simulink model "outerLoop_voltageControl"  (R2023b)
settings: Solver=ode1  StartTime=0.0  StopTime=Tsim_outLoop  FixedStep=Tstep  RelTol=1e-3
values from neighbouring files (symbols this model uses):
  C = 1000e-6    (= 0.001)    [DCDC_param.m]
  ILmax = 10    [DCDC_param.m]
  ILnom = 5    [DCDC_param.m]
  ResrC = 1.8e-3    (= 0.0018)    [DCDC_param.m]
  Tsw = 1/fsw    (= 0.0001)    [DCDC_param.m]    (also in adcpwm_setup.m)
  VinNom = 30    [DCDC_param.m]
  VoutNom = 50    [DCDC_param.m]
undefined symbols (not defined in the file or in its folder): den_i, kaw_v, ki_v, kp_v, kpf_v, num_i
settings Model: Creator=nicholas  LastModifiedBy=nicholas

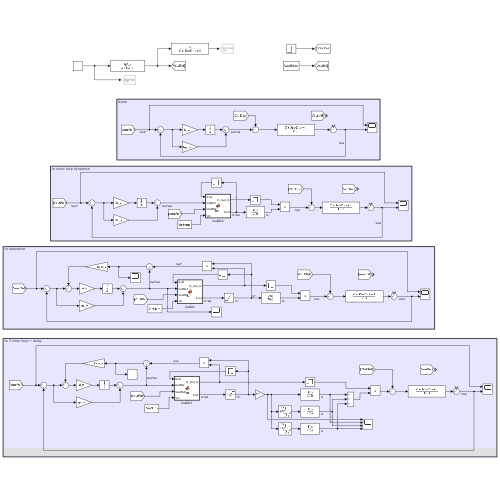
[thumbnail: Simulink's stored preview of the top-level diagram]
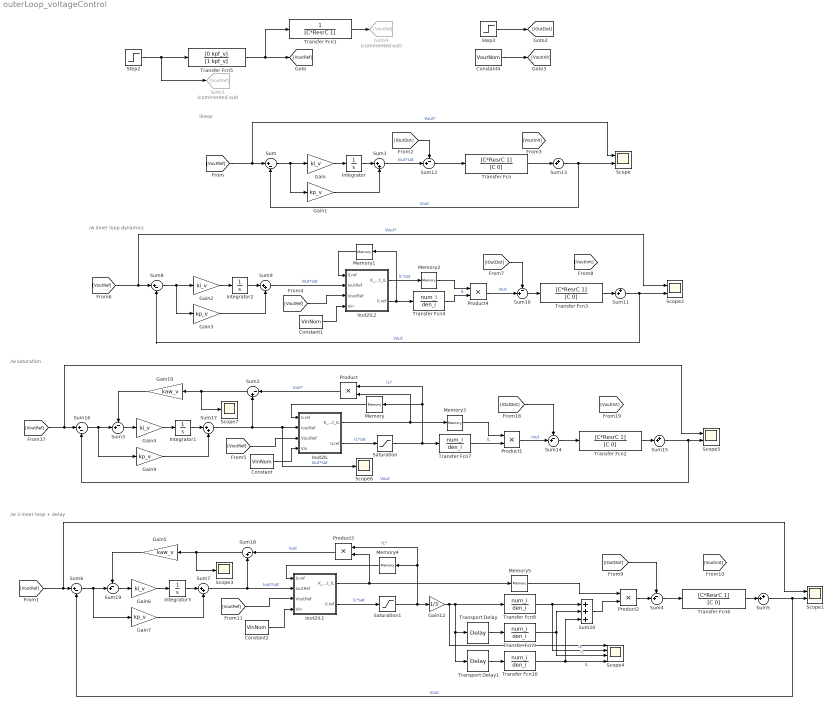
== system outerLoop_voltageControl ==
  note: /w 3 inner loop + delay
  note: /w saturation
  note: /w inner loop dynamics
  note: linear
  Constant : Constant  Value=VinNom
  Constant1 : Constant  Value=VinNom
  Constant2 : Constant  Value=VinNom
  Constant4 : Constant  Value=VoutNom
  Gain{,2,4,6} (4 alike) : Gain  Gain=ki_v
  Gain{1,3,7,9} (4 alike) : Gain  Gain=kp_v
  Gain10 : Gain  Gain=kaw_v
  Gain12 : Gain  Gain=1/3
  Gain5 : Gain  Gain=kaw_v
  Goto1 : Goto  Commented=on  GotoTag=VoutRef
  Goto4 : Goto  Commented=on  GotoTag=VoutRef
  Integrator{,1..3} (4 alike) : Integrator
  Iout2IL : MATLAB Function  TreatAsAtomicUnit=on
  Iout2IL1 : MATLAB Function  TreatAsAtomicUnit=on
  Iout2IL2 : MATLAB Function  TreatAsAtomicUnit=on
  Memory : Memory
  Memory1 : Memory
  Memory2 : Memory  InitialCondition=1
  Memory3 : Memory  InitialCondition=1
  Memory4 : Memory
  Memory5 : Memory  InitialCondition=1
  Product{,1..4} (5 alike) : Product
  Saturation : Saturate  UpperLimit=ILmax  LowerLimit=-ILmax
  Saturation1 : Saturate  UpperLimit=ILmax  LowerLimit=-ILmax
  Scope{,1..2,5} (4 alike) : Scope  NumInputPorts=2
  Scope3 : Scope
  Scope4 : Scope  NumInputPorts=4
  Scope6 : Scope
  Scope7 : Scope
  Step2 : Step  Time=0.1  Before=VinNom  After=VoutNom  SampleTime=0
  Step3 : Step  Time=0.3  After=ILnom/3  SampleTime=0
  Sum{,6,8,16} (4 alike) : Sum  Inputs=|+-
  Sum{1,7,9,17} (4 alike) : Sum  Inputs=|++
  Sum{3..4,10,12,14,19} (6 alike) : Sum  Inputs=-+|
  Sum{5,11,13,15} (4 alike) : Sum  Inputs=++|
  Sum18 : Sum  Inputs=|-+
  Sum2 : Sum  Inputs=|-+
  Sum20 : Sum  Inputs=+++
  Transfer Fcn{,2..3,6} (4 alike) : TransferFcn  Numerator=[C*ResrC 1]  Denominator=[C 0]
  Transfer Fcn1 : TransferFcn  Denominator=[C*ResrC 1]
  Transfer Fcn{4,7..10} (5 alike) : TransferFcn  Numerator=num_i  Denominator=den_i
  Transfer Fcn5 : TransferFcn  Numerator=[0 kpf_v]  Denominator=[1 kpf_v]
  Transport Delay : TransportDelay  DelayTime=Tsw/3
  Transport Delay1 : TransportDelay  DelayTime=2*Tsw/3
  wires:
  [VoutRef] -> Scope/1, Sum/1  "Vout*"
  Gain1/1 -> Sum1/2
  Sum/1 -> Gain/1, Gain1/1
  Gain/1 -> Integrator/1
  Integrator/1 -> Sum1/1
  Sum12/1 -> Transfer Fcn/1
  Step3/1 -> [IOutDist]
  Constant4/1 -> [VoutInit]
  Sum1/1 -> Sum12/2  "Iout*sat"
  Transfer Fcn/1 -> Sum13/2
  Sum13/1 -> Sum/2, Scope/2  "Vout"
  [IOutDist] -> Sum12/1
  Transfer Fcn1/1 -> Goto4/1
  Sum11/1 -> Sum8/2, Scope2/2  "Vout"
  Gain3/1 -> Sum9/2
  Transfer Fcn3/1 -> Sum11/2
  Sum8/1 -> Gain2/1, Gain3/1
  Sum10/1 -> Transfer Fcn3/1
  [VoutRef] -> Scope2/1, Sum8/1  "Vout*"
  Integrator2/1 -> Sum9/1
  [IOutDist] -> Sum10/1
  Gain2/1 -> Integrator2/1
  Product1/1 -> Sum14/2  "Iout"
  Gain9/1 -> Sum17/2
  Sum16/1 -> Sum3/2, Gain9/1
  Sum14/1 -> Transfer Fcn2/1
  Transfer Fcn2/1 -> Sum15/2
  Sum15/1 -> Sum16/2, Scope5/2  "Vout"
  [VoutRef] -> Scope5/1, Sum16/1
  Sum17/1 -> Sum2/2, Scope6/1, Iout2IL/2(IoutRef)  "Iout*sat"
  Integrator1/1 -> Sum17/1
  Sum3/1 -> Gain4/1
  Iout2IL/1(K_Iout_IL) -> Product/2, Memory3/1
  Memory/1 -> Iout2IL/1("ILref ")
  Constant/1 -> Iout2IL/4(Vin)
  Saturation/1 -> Transfer Fcn7/1, Product/1, Memory/1  "IL*"
  Sum9/1 -> Iout2IL2/2(IoutRef)  "Iout*sat"
  Iout2IL2/2(ILref) -> Memory1/1, Transfer Fcn4/1  "IL*sat"
  Memory1/1 -> Iout2IL2/1("ILref ")
  Constant1/1 -> Iout2IL2/4(Vin)
  [VoutRef] -> Iout2IL2/3(VoutRef)
  Product/1 -> Sum2/1  "Iout*"
  Sum2/1 -> Scope7/1, Gain10/1
  Transfer Fcn4/1 -> Product4/2  "IL"
  Product4/1 -> Sum10/2  "Iout"
  Iout2IL2/1(K_Iout_IL) -> Memory2/1
  Memory2/1 -> Product4/1
  Transfer Fcn7/1 -> Product1/2  "IL"
  Memory3/1 -> Product1/1
  Transfer Fcn5/1 -> Transfer Fcn1/1, [VoutRef]
  Step2/1 -> Transfer Fcn5/1, Goto1/1
  Gain4/1 -> Integrator1/1
  Gain10/1 -> Sum3/1
  [VoutRef] -> Iout2IL/3(VoutRef)
  Iout2IL/2(ILref) -> Saturation/1  "IL*sat"
  Integrator3/1 -> Sum7/1
  [VoutRef] -> Iout2IL1/3(VoutRef)
  Saturation1/1 -> Product3/1, Memory4/1, Gain12/1  "IL*"
  Gain6/1 -> Integrator3/1
  Sum7/1 -> Iout2IL1/2(IoutRef), Sum18/2  "Iout*sat"
  [IOutDist] -> Sum4/1
  Gain7/1 -> Sum7/2
  Sum4/1 -> Transfer Fcn6/1
  Iout2IL1/2(ILref) -> Saturation1/1  "IL*sat"
  Product2/1 -> Sum4/2
  Memory5/1 -> Product2/1
  Constant2/1 -> Iout2IL1/4(Vin)
  Sum6/1 -> Sum19/2, Gain7/1
  Iout2IL1/1(K_Iout_IL) -> Product3/2, Memory5/1
  Gain5/1 -> Sum19/1
  Sum5/1 -> Sum6/2, Scope1/2  "Vout"
  Sum19/1 -> Gain6/1
  Sum18/1 -> Scope3/1, Gain5/1
  Memory4/1 -> Iout2IL1/1("ILref ")
  [VoutRef] -> Scope1/1, Sum6/1
  Transfer Fcn6/1 -> Sum5/2
  Product3/1 -> Sum18/1  "Iout"
  Transport Delay/1 -> Transfer Fcn9/1
  Transport Delay1/1 -> Transfer Fcn10/1
  Gain12/1 -> Scope4/1, Transfer Fcn8/1, Transport Delay/1, Transport Delay1/1
  Transfer Fcn9/1 -> Scope4/3, Sum20/2  "IL"
  Transfer Fcn8/1 -> Scope4/2, Sum20/1  "IL"
  Transfer Fcn10/1 -> Scope4/4, Sum20/3  "IL"
  Sum20/1 -> Product2/2
  [IOutDist] -> Sum14/1

== matlab function outerLoop_voltageControl/Iout2IL1 ==
  data: K_Iout_IL output; ILref input; IoutRef input; VoutRef input; Vin input; ILref output; RserL parameter
function [K_Iout_IL,ILref] = fcn(ILref,IoutRef,VoutRef,Vin,RserL)

if VoutRef < Vin
    VoutRef = Vin;
end
K_Iout_IL = (Vin - RserL*ILref) / VoutRef;
ILref = IoutRef / K_Iout_IL;

== matlab function outerLoop_voltageControl/Iout2IL2 ==
  data: K_Iout_IL output; ILref input; IoutRef input; VoutRef input; Vin input; ILref output; RserL parameter
function [K_Iout_IL,ILref] = fcn(ILref,IoutRef,VoutRef,Vin,RserL)

if VoutRef < Vin
    VoutRef = Vin;
end
K_Iout_IL = (Vin - RserL*ILref) / VoutRef;
ILref = IoutRef / K_Iout_IL;

== matlab function outerLoop_voltageControl/Iout2IL ==
  data: K_Iout_IL output; ILref input; IoutRef input; VoutRef input; Vin input; ILref output; RserL parameter
function [K_Iout_IL,ILref] = fcn(ILref,IoutRef,VoutRef,Vin,RserL)

if VoutRef < Vin
    VoutRef = Vin;
end
K_Iout_IL = (Vin - RserL*ILref) / VoutRef;
ILref = IoutRef / K_Iout_IL;
